simulink model "torqueBalancingJc"  (Simulink 8.6)
settings: Solver=FixedStepDiscrete  StartTime=0.0  StopTime=simulationTime  FixedStep=Ts  RelTol=1e-3
InitFcn:
  | initTorqueBalancingJc;
values from neighbouring files (symbols this model uses):
  LEFT_RIGHT_FOOT_IN_CONTACT = [1 1]    [initTorqueBalancingJc.m]
  localName = 'matlabTorqueBalancing'    [initTorqueBalancingJc.m]
  Ts = 0.01    [initTorqueBalancingJc.m]
undefined symbols (not defined in the file or in its folder): bVectorConstraints, ConstraintsMatrix, gain, impedencesSat, reg, ROBOT_DOF, ROBOT_DOF_FOR_SIMULINK, sat
undefined symbols (not defined in the file): robotName
libraries: WBCLibrary x63, simulink x2
settings Model: Creator=daniele  LastModifiedBy=DanielePucci
settings DataIOCC: SignalLoggingSaveFormat=Dataset
settings DebuggingCC: FcnCallInpInsideContextMsg=EnableAllAsWarning
settings SFSimCC: SimParseCustomCode=off
settings ConfigComp: CovSFcnEnable=off

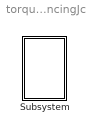
== system torqueBalancingJc ==
  Subsystem : Subsystem  mask{robotName=robotName, Ts=Ts, localName=localName}
      mask prompts: robotName "robot name"; localName "module name"

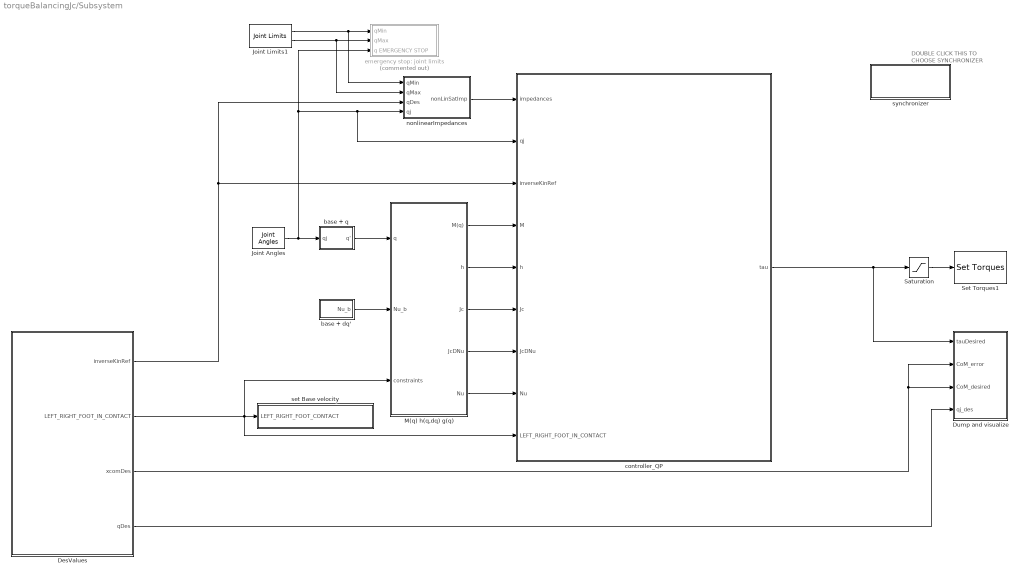
== system torqueBalancingJc/Subsystem ==
  note: DOUBLE CLICK THIS TO
      |  CHOOSE SYNCHRONIZER
  DesValues : Subsystem
  Dump and visualize : Subsystem
  Joint Angles : WBCLibrary/wholeBodyStates/Joint Angles  robotName=robotName  localName=localName
  Joint Limits1 : WBCLibrary/wholeBodyModel/Joint Limits  robotName=robotName  localName=localName
  M(q) h(q,dq) g(q) : Subsystem
  Saturation : Saturate  UpperLimit=sat.torque  LowerLimit=-sat.torque
  Set Torques1 : WBCLibrary/wholeBodyActuators/Set Torques  val=6  robotName=robotName  localName=localName
  base + dq' : Subsystem
  base + q : Subsystem
  controller_QP : Subsystem
  emergency stop: joint limits : Subsystem  Commented=on
  nonlinearImpedances : Subsystem
  set Base velocity : Subsystem  Description=Set base velocity
  synchronizer : Subsystem
  wires:
  base + q/1(q') -> M(q) h(q,dq) g(q)/1(q)
  base + dq'/1(Nu_b) -> M(q) h(q,dq) g(q)/2(Nu_b)
  M(q) h(q,dq) g(q)/1(M(q)) -> controller_QP/4(M)
  Joint Limits1/1 -> emergency stop: joint limits/1(qMin), nonlinearImpedances/1(qMin)
  Joint Limits1/2 -> emergency stop: joint limits/2(qMax), nonlinearImpedances/2(qMax)
  Joint Angles/1 -> emergency stop: joint limits/3(q EMERGENCY STOP), controller_QP/2(qj), nonlinearImpedances/4(qj), base + q/1(qj)
  M(q) h(q,dq) g(q)/2(h) -> controller_QP/5(h)
  controller_QP/1("tau ") -> Dump and visualize/1(tauDesired), Saturation/1
  Saturation/1 -> Set Torques1/1
  DesValues/2(LEFT_RIGHT_FOOT_IN_CONTACT) -> M(q) h(q,dq) g(q)/3(constraints), set Base velocity/1(LEFT_RIGHT_FOOT_CONTACT), controller_QP/9(LEFT_RIGHT_FOOT_IN_CONTACT)
  DesValues/3(xcomDes) -> Dump and visualize/2(CoM_error), Dump and visualize/3(CoM_desired)
  nonlinearImpedances/1(nonLinSatImp) -> controller_QP/1(impedances)
  M(q) h(q,dq) g(q)/5(Nu) -> controller_QP/8(Nu)
  M(q) h(q,dq) g(q)/3(Jc) -> controller_QP/6(Jc)
  M(q) h(q,dq) g(q)/4(JcDNu) -> controller_QP/7(JcDNu)
  DesValues/1(inverseKinRef) -> nonlinearImpedances/3(qDes), controller_QP/3(inverseKinRef)
  DesValues/4(qDes) -> Dump and visualize/4(qj_des)

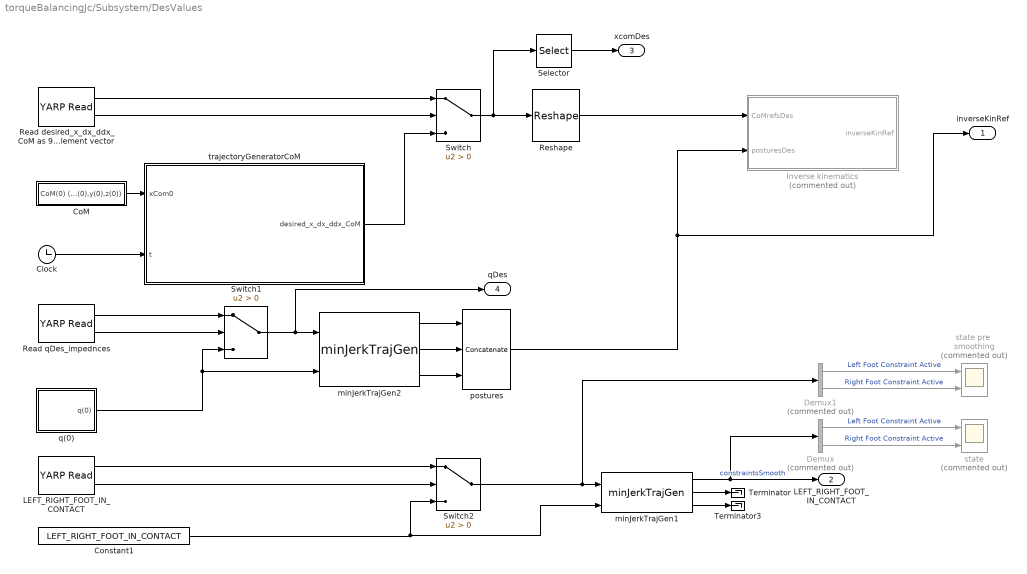
== system torqueBalancingJc/Subsystem/DesValues ==
  " LEFT_RIGHT_FOOT_IN_CONTACT" : WBCLibrary/Utilities/YARP Read  portName=['/' localName '/constraints:i']  signalSize=2  blocking=off  timestamp=off  autoconnect=off  errorOnConnection=on
  Clock : Clock
  "CoM " : Subsystem
  Constant1 : Constant  Value=LEFT_RIGHT_FOOT_IN_CONTACT
  Demux : Demux  Commented=on  Outputs=2
  Demux1 : Demux  Commented=on  Outputs=2
  Inverse kinematics : Subsystem  Commented=on
  "Read desired_x_dx_ddx_CoM as 9 element vector " : WBCLibrary/Utilities/YARP Read  portName=['/' localName '/comDes:i']  signalSize=9  blocking=off  timestamp=off  autoconnect=off  errorOnConnection=on
  Read qDes_impednces : WBCLibrary/Utilities/YARP Read  portName=['/' localName '/qDes:i']  signalSize=ROBOT_DOF  blocking=off  timestamp=off  autoconnect=off  errorOnConnection=on
  Reshape : Reshape  OutputDimensionality=Customize  OutputDimensions=[3,3]
  Selector : Selector  InputPortWidth=9  IndexOptions=Index vector (dialog)  Indices=[1:3]  OutputSizes=1
  Switch : Switch  Criteria=u2 > Threshold
  Switch1 : Switch  Criteria=u2 > Threshold
  Switch2 : Switch  Criteria=u2 > Threshold
  Terminator : Terminator
  Terminator3 : Terminator
  minJerkTrajGen1 : WBCLibrary/Utilities/minJerkTrajGen  dim=2  Ts=Ts  Tt=smoothingTimeJacobians
  minJerkTrajGen2 : WBCLibrary/Utilities/minJerkTrajGen  dim=ROBOT_DOF  Ts=Ts  Tt=smoothingTimePostures
  postures : Concatenate  NumInputs=3  Mode=Multidimensional array  ConcatenateDimension=2
  q(0) : Subsystem
  state : Scope  Commented=on  NumInputPorts=2
  state pre  smoothing : Scope  Commented=on  NumInputPorts=2
  trajectoryGeneratorCoM : MATLAB Function  TreatAsAtomicUnit=on
  inverseKinRef : Outport
  LEFT_RIGHT_FOOT_IN_CONTACT : Outport  Port=2
  xcomDes : Outport  Port=3
  qDes : Outport  Port=4
  wires:
  Constant1/1 -> minJerkTrajGen1/2, Switch2/3
  minJerkTrajGen1/1 -> Demux/1, LEFT_RIGHT_FOOT_IN_CONTACT/1  "constraintsSmooth"
  minJerkTrajGen1/2 -> Terminator/1
  minJerkTrajGen1/3 -> Terminator3/1
  "Read desired_x_dx_ddx_CoM as 9 element vector "/2 -> Switch/2
  "Read desired_x_dx_ddx_CoM as 9 element vector "/1 -> Switch/1
  Reshape/1 -> Inverse kinematics/1(CoMrefsDes)
  Switch/1 -> Selector/1, Reshape/1
  Read qDes_impednces/2 -> Switch1/2
  Read qDes_impednces/1 -> Switch1/1
  q(0)/1(q(0)) -> Switch1/3, minJerkTrajGen2/2
  Selector/1 -> xcomDes/1
  " LEFT_RIGHT_FOOT_IN_CONTACT"/2 -> Switch2/2
  " LEFT_RIGHT_FOOT_IN_CONTACT"/1 -> Switch2/1
  Switch2/1 -> Demux1/1, minJerkTrajGen1/1
  Demux/1 -> state/1  "Left Foot Constraint Active"
  Demux/2 -> state/2  "Right Foot Constraint Active"
  Demux1/1 -> state pre  smoothing/1  "Left Foot Constraint Active"
  Demux1/2 -> state pre  smoothing/2  "Right Foot Constraint Active"
  "CoM "/1(CoM(0) (x(0),y(0),z(0))) -> trajectoryGeneratorCoM/1(xCom0)
  Clock/1 -> trajectoryGeneratorCoM/2(t)
  trajectoryGeneratorCoM/1(desired_x_dx_ddx_CoM) -> Switch/3
  Switch1/1 -> qDes/1, minJerkTrajGen2/1
  minJerkTrajGen2/1 -> postures/1
  minJerkTrajGen2/2 -> postures/2
  minJerkTrajGen2/3 -> postures/3
  postures/1 -> inverseKinRef/1, Inverse kinematics/2(posturesDes)

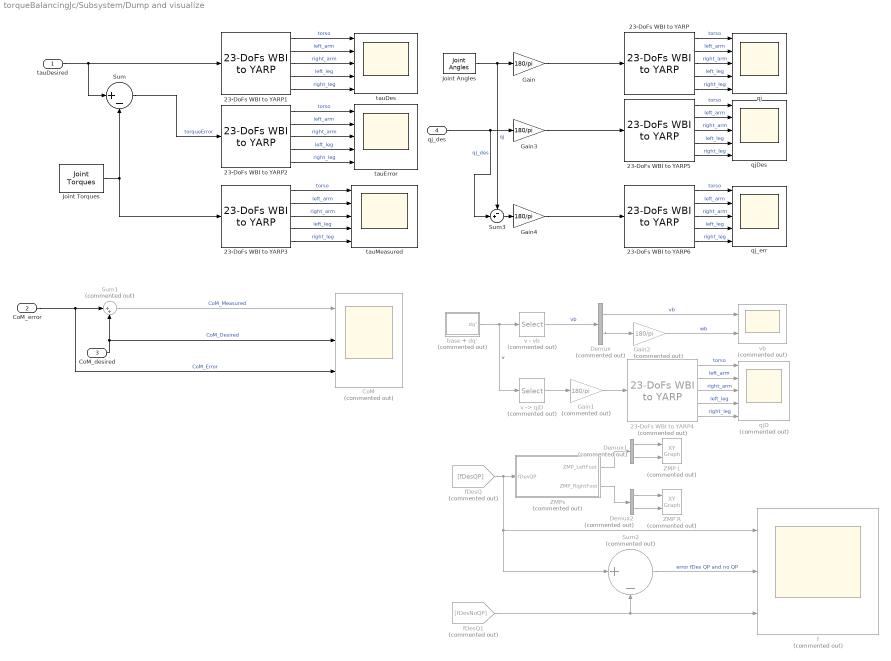
== system torqueBalancingJc/Subsystem/Dump and visualize ==
  tauDesired : Inport
  CoM_error : Inport  Port=2
  CoM_desired : Inport  Port=3
  qj_des : Inport  Port=4
  23-DoFs WBI to YARP{,1..3,5..6} (6 alike) : WBCLibrary/Utilities/23-DoFs WBI to YARP
  23-DoFs WBI to YARP4 : WBCLibrary/Utilities/23-DoFs WBI to YARP  Commented=on
  CoM : Scope  Commented=on  NumInputPorts=3
  Demux : Demux  Commented=on  Outputs=2
  Demux1 : Demux  Commented=on  Outputs=2
  Demux2 : Demux  Commented=on  Outputs=2
  Gain : Gain  Gain=180/pi
  Gain1 : Gain  Commented=on  Gain=180/pi
  Gain2 : Gain  Commented=on  Gain=180/pi
  Gain3 : Gain  Gain=180/pi
  Gain4 : Gain  Gain=180/pi
  Joint Angles : WBCLibrary/wholeBodyStates/Joint Angles  robotName=robotName  localName=localName
  Joint Torques : WBCLibrary/wholeBodyStates/Joint Torques  robotName=robotName  localName=localName
  Sum : Sum  Inputs=|+-
  Sum1 : Sum  Commented=on  Inputs=|++
  Sum2 : Sum  Commented=on  Inputs=|+-
  Sum3 : Sum  Inputs=-+|
  ZMP L : simulink/Sinks/XY Graph  Commented=on  xmin=gain.footSize(1,1)  xmax=gain.footSize(1,2)  ymin=gain.footSize(2,1)  ymax=gain.footSize(2,2)  st=-1
  ZMP R : simulink/Sinks/XY Graph  Commented=on  xmin=gain.footSize(1,1)  xmax=gain.footSize(1,2)  ymin=gain.footSize(2,1)  ymax=gain.footSize(2,2)  st=-1
  ZMPs : Subsystem  Commented=on
  base + dq' : Subsystem  Commented=on
  f : Scope  Commented=on  NumInputPorts=3
  fDesQ : From  Commented=on  GotoTag=fDesQP  TagVisibility=global
  fDesQ1 : From  Commented=on  GotoTag=fDesNoQP  TagVisibility=global
  qj : Scope  NumInputPorts=5
  qjD : Scope  Commented=on  NumInputPorts=5
  qjDes : Scope  NumInputPorts=5
  qj_err : Scope  NumInputPorts=5
  tauDes : Scope  NumInputPorts=5
  tauError : Scope  NumInputPorts=5
  tauMeasured : Scope  NumInputPorts=5
  v - vb : Selector  Commented=on  InputPortWidth=ROBOT_DOF+6  IndexOptions=Index vector (dialog)  Indices=[1:6]  OutputSizes=1
  "v -> qjD" : Selector  Commented=on  InputPortWidth=ROBOT_DOF+6  IndexOptions=Index vector (dialog)  Indices=[7:ROBOT_DOF+6]  OutputSizes=1
  vb : Scope  Commented=on  NumInputPorts=2
  wires:
  CoM_error/1 -> CoM/3, Sum1/1  "CoM_Error"
  CoM_desired/1 -> Sum1/2, CoM/2  "CoM_Desired"
  Sum1/1 -> CoM/1  "CoM_Measured"
  base + dq'/1(dq') -> "v -> qjD"/1, v - vb/1  "v"
  Joint Angles/1 -> Sum3/1, Gain/1  "qj"
  Gain/1 -> 23-DoFs WBI to YARP/1
  23-DoFs WBI to YARP/5 -> qj/5  "right_leg"
  23-DoFs WBI to YARP/1 -> qj/1  "torso"
  23-DoFs WBI to YARP/2 -> qj/2  "left_arm"
  23-DoFs WBI to YARP/4 -> qj/4  "left_leg"
  23-DoFs WBI to YARP/3 -> qj/3  "right_arm"
  23-DoFs WBI to YARP4/5 -> qjD/5  "right_leg"
  23-DoFs WBI to YARP4/1 -> qjD/1  "torso"
  23-DoFs WBI to YARP4/2 -> qjD/2  "left_arm"
  23-DoFs WBI to YARP4/4 -> qjD/4  "left_leg"
  23-DoFs WBI to YARP4/3 -> qjD/3  "right_arm"
  "v -> qjD"/1 -> Gain1/1
  v - vb/1 -> Demux/1  "vb"
  Demux/1 -> vb/1  "vb"
  Demux/2 -> Gain2/1
  Gain1/1 -> 23-DoFs WBI to YARP4/1
  Gain2/1 -> vb/2  "wb"
  fDesQ/1 -> Sum2/1, f/1, ZMPs/1(fDesQP)
  ZMPs/1(ZMP_LeftFoot) -> Demux1/1
  ZMPs/2(ZMP_RightFoot) -> Demux2/1
  Demux1/1 -> ZMP L/1
  Demux1/2 -> ZMP L/2
  Demux2/1 -> ZMP R/1
  Demux2/2 -> ZMP R/2
  Sum2/1 -> f/2  "error fDes QP and no QP"
  fDesQ1/1 -> Sum2/2, f/3
  tauDesired/1 -> Sum/1, 23-DoFs WBI to YARP1/1
  Joint Torques/1 -> 23-DoFs WBI to YARP3/1, Sum/2
  23-DoFs WBI to YARP1/5 -> tauDes/5  "right_leg"
  23-DoFs WBI to YARP1/1 -> tauDes/1  "torso"
  23-DoFs WBI to YARP1/2 -> tauDes/2  "left_arm"
  23-DoFs WBI to YARP1/4 -> tauDes/4  "left_leg"
  23-DoFs WBI to YARP1/3 -> tauDes/3  "right_arm"
  23-DoFs WBI to YARP2/5 -> tauError/5  "right_leg"
  23-DoFs WBI to YARP2/1 -> tauError/1  "torso"
  23-DoFs WBI to YARP2/2 -> tauError/2  "left_arm"
  23-DoFs WBI to YARP2/4 -> tauError/4  "left_leg"
  23-DoFs WBI to YARP2/3 -> tauError/3  "right_arm"
  Sum/1 -> 23-DoFs WBI to YARP2/1  "torqueError"
  23-DoFs WBI to YARP3/5 -> tauMeasured/5  "right_leg"
  23-DoFs WBI to YARP3/1 -> tauMeasured/1  "torso"
  23-DoFs WBI to YARP3/2 -> tauMeasured/2  "left_arm"
  23-DoFs WBI to YARP3/4 -> tauMeasured/4  "left_leg"
  23-DoFs WBI to YARP3/3 -> tauMeasured/3  "right_arm"
  Gain3/1 -> 23-DoFs WBI to YARP5/1
  23-DoFs WBI to YARP5/5 -> qjDes/5  "right_leg"
  23-DoFs WBI to YARP5/1 -> qjDes/1  "torso"
  23-DoFs WBI to YARP5/2 -> qjDes/2  "left_arm"
  23-DoFs WBI to YARP5/4 -> qjDes/4  "left_leg"
  23-DoFs WBI to YARP5/3 -> qjDes/3  "right_arm"
  Gain4/1 -> 23-DoFs WBI to YARP6/1
  23-DoFs WBI to YARP6/5 -> qj_err/5  "right_leg"
  23-DoFs WBI to YARP6/1 -> qj_err/1  "torso"
  23-DoFs WBI to YARP6/2 -> qj_err/2  "left_arm"
  23-DoFs WBI to YARP6/4 -> qj_err/4  "left_leg"
  23-DoFs WBI to YARP6/3 -> qj_err/3  "right_arm"
  Sum3/1 -> Gain4/1
  qj_des/1 -> Sum3/2, Gain3/1  "qj_des"

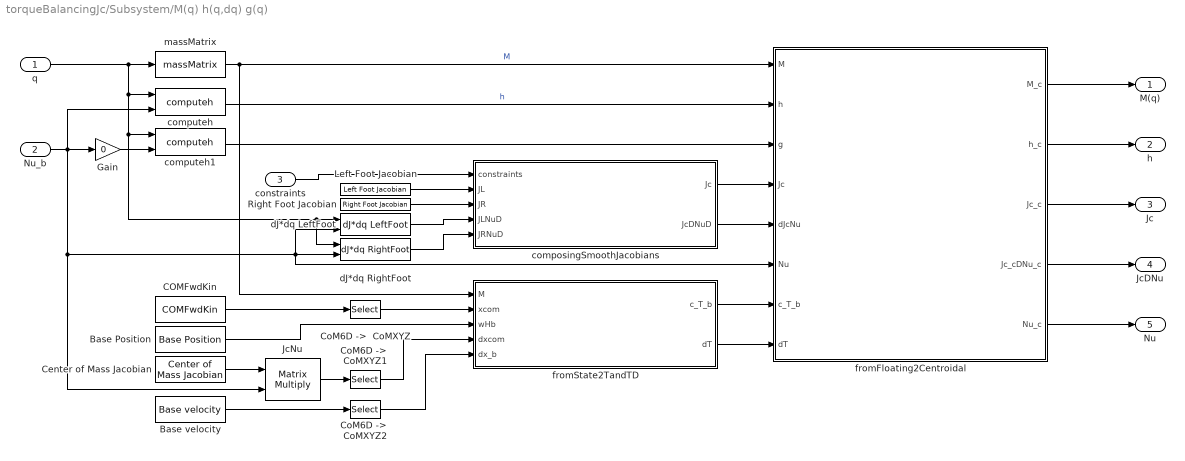
== system torqueBalancingJc/Subsystem/M(q) h(q,dq) g(q) ==
  q : Inport
  Nu_b : Inport  Port=2
  constraints : Inport  Port=3
  Base Position : WBCLibrary/wholeBodyStates/Base Position  robotName=robotName  localName=localName
  Base velocity : WBCLibrary/wholeBodyStates/Base velocity  robotName=robotName  localName=localName
  "COMFwdKin " : WBCLibrary/wholeBodyModel/Forward Kinematics/COMFwdKin   robotName=robotName  localName=localName
  Center of Mass Jacobian : WBCLibrary/wholeBodyModel/Jacobians/Center of Mass Jacobian  robotName=robotName  localName=localName
  "CoM6D ->  CoMXYZ" : Selector  InputPortWidth=7  IndexOptions=Index vector (dialog)  Indices=[1 2 3]  OutputSizes=1
  "CoM6D ->  CoMXYZ1" : Selector  InputPortWidth=6  IndexOptions=Index vector (dialog)  Indices=[1 2 3]  OutputSizes=1
  "CoM6D ->  CoMXYZ2" : Selector  InputPortWidth=6  IndexOptions=Index vector (dialog)  Indices=[1 2 3]  OutputSizes=1
  Gain : Gain  Gain=0
  JcNu : Product  Multiplication=Matrix(*)
  Left Foot Jacobian : WBCLibrary/wholeBodyModel/Jacobians/Left Foot Jacobian  robotName=robotName  localName=localName
  Right Foot Jacobian : WBCLibrary/wholeBodyModel/Jacobians/Right Foot Jacobian  robotName=robotName  localName=localName
  composingSmoothJacobians : MATLAB Function  TreatAsAtomicUnit=on
  computeh : WBCLibrary/wholeBodyModel/Dynamics/computeh  val=7  robotname=robotName  localname=localName
  computeh1 : WBCLibrary/wholeBodyModel/Dynamics/computeh  val=7  robotname=robotName  localname=localName
  dJ*dq LeftFoot : WBCLibrary/wholeBodyModel/Dynamics/dJ*dq LeftFoot  val=9  robotName=robotName  localName=localName
  dJ*dq RightFoot : WBCLibrary/wholeBodyModel/Dynamics/dJ*dq RightFoot  val=9  robotName=robotName  localName=localName
  fromFloating2Centroidal : MATLAB Function  TreatAsAtomicUnit=on
  fromState2TandTD : MATLAB Function  TreatAsAtomicUnit=on
  massMatrix : WBCLibrary/wholeBodyModel/Dynamics/massMatrix  val=8  robotname=robotName  localname=localName
  M(q) : Outport
  h : Outport  Port=2
  Jc : Outport  Port=3
  JcDNu : Outport  Port=4
  Nu : Outport  Port=5
  wires:
  q/1 -> computeh1/1, dJ*dq RightFoot/1, dJ*dq LeftFoot/1, computeh/1, massMatrix/1
  Nu_b/1 -> Gain/1, computeh/2, fromFloating2Centroidal/6(Nu), dJ*dq LeftFoot/2, dJ*dq RightFoot/2, JcNu/2
  Gain/1 -> computeh1/2
  massMatrix/1 -> fromFloating2Centroidal/1(M), fromState2TandTD/1(M)  "M"
  fromState2TandTD/1(c_T_b) -> fromFloating2Centroidal/7(c_T_b)
  fromState2TandTD/2(dT) -> fromFloating2Centroidal/8(dT)
  computeh/1 -> fromFloating2Centroidal/2(h)  "h"
  computeh1/1 -> fromFloating2Centroidal/3(g)
  "COMFwdKin "/1 -> "CoM6D ->  CoMXYZ"/1
  "CoM6D ->  CoMXYZ"/1 -> fromState2TandTD/2(xcom)
  Base velocity/1 -> "CoM6D ->  CoMXYZ2"/1
  "CoM6D ->  CoMXYZ2"/1 -> fromState2TandTD/5(dx_b)
  Base Position/1 -> fromState2TandTD/3(wHb)
  Center of Mass Jacobian/1 -> JcNu/1
  JcNu/1 -> "CoM6D ->  CoMXYZ1"/1
  "CoM6D ->  CoMXYZ1"/1 -> fromState2TandTD/4(dxcom)
  composingSmoothJacobians/1(Jc) -> fromFloating2Centroidal/4(Jc)
  composingSmoothJacobians/2(JcDNuD) -> fromFloating2Centroidal/5(dJcNu)
  constraints/1 -> composingSmoothJacobians/1(constraints)
  Left Foot Jacobian/1 -> composingSmoothJacobians/2(JL)
  Right Foot Jacobian/1 -> composingSmoothJacobians/3(JR)
  dJ*dq LeftFoot/1 -> composingSmoothJacobians/4(JLNuD)
  dJ*dq RightFoot/1 -> composingSmoothJacobians/5(JRNuD)
  fromFloating2Centroidal/1(M_c) -> M(q)/1
  fromFloating2Centroidal/2(h_c) -> h/1
  fromFloating2Centroidal/3(Jc_c) -> Jc/1
  fromFloating2Centroidal/4(Jc_cDNu_c) -> JcDNu/1
  fromFloating2Centroidal/5(Nu_c) -> Nu/1

== system torqueBalancingJc/Subsystem/base + dq' ==
  Base velocity : WBCLibrary/wholeBodyStates/Base velocity  robotName=robotName  localName=localName
  Joint Velocities : WBCLibrary/wholeBodyStates/Joint Velocities  robotName=robotName  localName=localName
  Mux : Mux  Inputs=2
  Nu_b : Outport
  wires:
  Base velocity/1 -> Mux/1
  Joint Velocities/1 -> Mux/2
  Mux/1 -> Nu_b/1

== system torqueBalancingJc/Subsystem/base + q ==
  qj : Inport
  Constant1 : Constant  Value=zeros(16,1)
  Mux : Mux  Inputs=2
  q' : Outport
  wires:
  Mux/1 -> q'/1
  qj/1 -> Mux/2
  Constant1/1 -> Mux/1

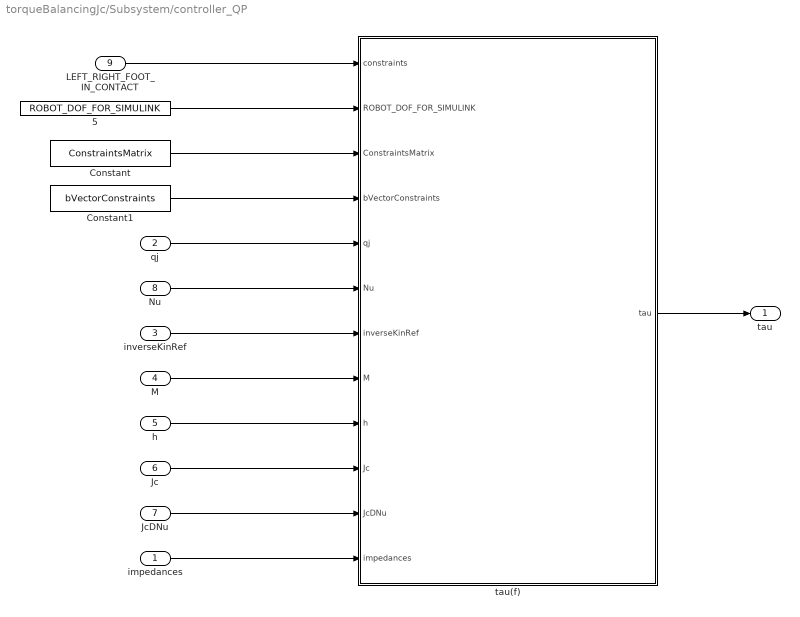
== system torqueBalancingJc/Subsystem/controller_QP ==
  impedances : Inport
  qj : Inport  Port=2
  inverseKinRef : Inport  Port=3
  M : Inport  Port=4
  h : Inport  Port=5
  Jc : Inport  Port=6
  JcDNu : Inport  Port=7
  Nu : Inport  Port=8
  LEFT_RIGHT_FOOT_IN_CONTACT : Inport  Port=9
  "    5" : Constant  Value=ROBOT_DOF_FOR_SIMULINK
  Constant : Constant  Value=ConstraintsMatrix
  Constant1 : Constant  Value=bVectorConstraints
  "tau(f) " : MATLAB Function  TreatAsAtomicUnit=on
  "tau " : Outport
  wires:
  LEFT_RIGHT_FOOT_IN_CONTACT/1 -> "tau(f) "/1(constraints)
  M/1 -> "tau(f) "/8(M)
  h/1 -> "tau(f) "/9(h)
  "    5"/1 -> "tau(f) "/2(ROBOT_DOF_FOR_SIMULINK)
  Constant/1 -> "tau(f) "/3(ConstraintsMatrix)
  Constant1/1 -> "tau(f) "/4(bVectorConstraints)
  Jc/1 -> "tau(f) "/10(Jc)
  JcDNu/1 -> "tau(f) "/11(JcDNu)
  Nu/1 -> "tau(f) "/6(Nu)
  impedances/1 -> "tau(f) "/12(impedances)
  "tau(f) "/1(tau) -> "tau "/1
  qj/1 -> "tau(f) "/5(qj)
  inverseKinRef/1 -> "tau(f) "/7(inverseKinRef)

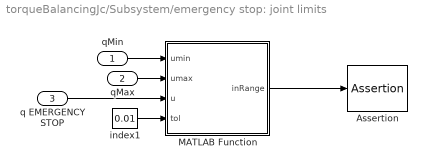
== system torqueBalancingJc/Subsystem/emergency stop: joint limits ==
  qMin : Inport
  qMax : Inport  Port=2
  q EMERGENCY STOP : Inport  Port=3
  Assertion : Assertion
  MATLAB Function : MATLAB Function  TreatAsAtomicUnit=on
  index1 : Constant  Value=0.01  VectorParams1D=off
  wires:
  qMin/1 -> MATLAB Function/1(umin)
  qMax/1 -> MATLAB Function/2(umax)
  index1/1 -> MATLAB Function/4(tol)
  q EMERGENCY STOP/1 -> MATLAB Function/3(u)
  MATLAB Function/1(inRange) -> Assertion/1

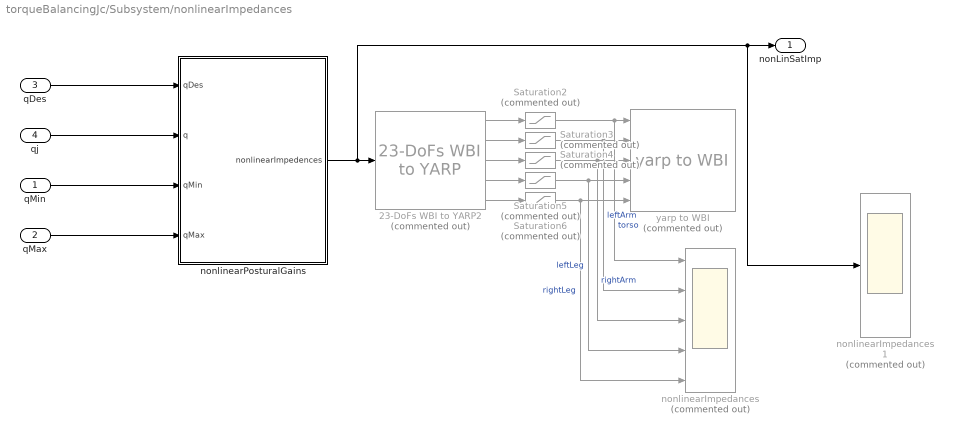
== system torqueBalancingJc/Subsystem/nonlinearImpedances ==
  qMin : Inport
  qMax : Inport  Port=2
  qDes : Inport  Port=3
  qj : Inport  Port=4
  23-DoFs WBI to YARP2 : WBCLibrary/Utilities/23-DoFs WBI to YARP  Commented=on
  Saturation2 : Saturate  Commented=on  UpperLimit=impedencesSat(1)  LowerLimit=0  SampleTime=Ts
  Saturation3 : Saturate  Commented=on  UpperLimit=impedencesSat(2)  LowerLimit=0  SampleTime=Ts
  Saturation4 : Saturate  Commented=on  UpperLimit=impedencesSat(2)  LowerLimit=0  SampleTime=Ts
  Saturation5 : Saturate  Commented=on  UpperLimit=impedencesSat(3)  LowerLimit=0  SampleTime=Ts
  Saturation6 : Saturate  Commented=on  UpperLimit=impedencesSat(3)  LowerLimit=0  SampleTime=Ts
  nonlinearImpedances : Scope  Commented=on  NumInputPorts=5
  nonlinearImpedances1 : Scope  Commented=on
  "nonlinearPosturalGains " : MATLAB Function  TreatAsAtomicUnit=on
  yarp to WBI : WBCLibrary/Utilities/yarp to WBI  Commented=on
  nonLinSatImp : Outport
  wires:
  23-DoFs WBI to YARP2/1 -> Saturation2/1
  23-DoFs WBI to YARP2/2 -> Saturation3/1
  23-DoFs WBI to YARP2/3 -> Saturation4/1
  23-DoFs WBI to YARP2/5 -> Saturation6/1
  "nonlinearPosturalGains "/1(nonlinearImpedences) -> nonlinearImpedances1/1, nonLinSatImp/1, 23-DoFs WBI to YARP2/1
  qMin/1 -> "nonlinearPosturalGains "/3(qMin)
  qMax/1 -> "nonlinearPosturalGains "/4(qMax)
  qj/1 -> "nonlinearPosturalGains "/2(q)
  Saturation6/1 -> nonlinearImpedances/5, yarp to WBI/5  "rightLeg"
  Saturation4/1 -> nonlinearImpedances/3, yarp to WBI/3  "rightArm"
  Saturation5/1 -> nonlinearImpedances/4, yarp to WBI/4  "leftLeg"
  Saturation3/1 -> nonlinearImpedances/2, yarp to WBI/2  "leftArm"
  Saturation2/1 -> nonlinearImpedances/1, yarp to WBI/1  "torso"
  23-DoFs WBI to YARP2/4 -> Saturation5/1
  qDes/1 -> "nonlinearPosturalGains "/1(qDes)

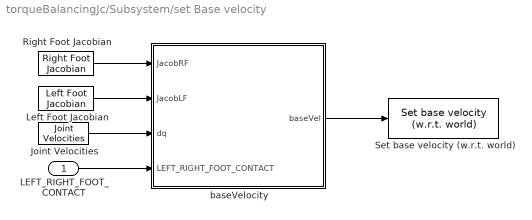
== system torqueBalancingJc/Subsystem/set Base velocity ==
  LEFT_RIGHT_FOOT_CONTACT : Inport
  Joint Velocities : WBCLibrary/wholeBodyStates/Joint Velocities  robotName=robotName  localName=localName
  Left Foot Jacobian : WBCLibrary/wholeBodyModel/Jacobians/Left Foot Jacobian  robotName=robotName  localName=localName
  Right Foot Jacobian : WBCLibrary/wholeBodyModel/Jacobians/Right Foot Jacobian  robotName=robotName  localName=localName
  Set base velocity (w.r.t. world) : WBCLibrary/wholeBodyStates/Set base velocity (w.r.t. world)  Priority=-1  robotName=robotName  localName=localName
  baseVelocity : Subsystem  AncestorBlock=WBCLibrary/Utilities/baseVelocity  mask(baseVelocity){}
      mask help: This block computes the velocity of the floating base of a bipedal robot
  wires:
  Left Foot Jacobian/1 -> baseVelocity/2(JacobLF)
  Right Foot Jacobian/1 -> baseVelocity/1(JacobRF)
  baseVelocity/1(baseVel) -> Set base velocity (w.r.t. world)/1
  Joint Velocities/1 -> baseVelocity/3(dq)
  LEFT_RIGHT_FOOT_CONTACT/1 -> baseVelocity/4(LEFT_RIGHT_FOOT_CONTACT)

== system torqueBalancingJc/Subsystem/synchronizer ==
  Real Time Synchronizer : WBCLibrary/Utilities/Real Time Synchronizer  threadPeriod=Ts
  synchronize : WBCLibrary/Utilities/synchronize  Commented=on  rate=0.010  scaleFactor=1

== system torqueBalancingJc/Subsystem/DesValues/CoM  ==
  "COMFwdKin " : WBCLibrary/wholeBodyModel/Forward Kinematics/COMFwdKin   robotName=robotName  localName=localName
  "CoM6D ->  CoMXYZ" : Selector  InputPortWidth=7  IndexOptions=Index vector (dialog)  Indices=[1 2 3]  OutputSizes=1
  "holder " : WBCLibrary/Utilities/holder 
  CoM(0) (x(0),y(0),z(0)) : Outport
  wires:
  "COMFwdKin "/1 -> "CoM6D ->  CoMXYZ"/1
  "CoM6D ->  CoMXYZ"/1 -> "holder "/1
  "holder "/1 -> CoM(0) (x(0),y(0),z(0))/1

== system torqueBalancingJc/Subsystem/DesValues/Inverse kinematics ==
  CoMrefsDes : Inport
  posturesDes : Inport  Port=2
  base + dq' : Subsystem
  iKin Stack of Tasks : Subsystem
  iKin correction terms : Subsystem
  inverseKinRef : Outport
  wires:
  CoMrefsDes/1 -> iKin correction terms/1(CoMrefsDes)
  posturesDes/1 -> iKin correction terms/2(posturesDes)
  base + dq'/1(Nu_b) -> iKin correction terms/4(Nu_iKin)

== system torqueBalancingJc/Subsystem/DesValues/q(0) ==
  Joint Angles : WBCLibrary/wholeBodyStates/Joint Angles  robotName=robotName  localName=localName
  holder 1 : WBCLibrary/Utilities/holder 
  q(0) : Outport
  wires:
  Joint Angles/1 -> holder 1/1
  holder 1/1 -> q(0)/1

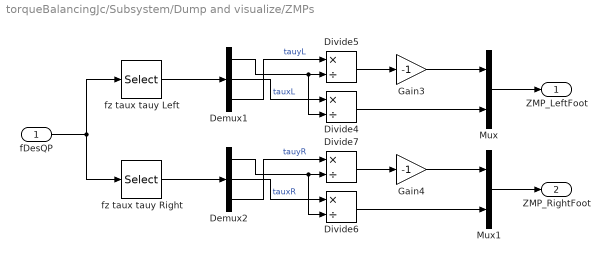
== system torqueBalancingJc/Subsystem/Dump and visualize/ZMPs ==
  fDesQP : Inport
  Demux1 : Demux  Outputs=3
  Demux2 : Demux  Outputs=3
  Divide{4..7} (4 alike) : Product  Inputs=*/
  Gain3 : Gain  Gain=-1
  Gain4 : Gain  Gain=-1
  Mux : Mux  Inputs=2
  Mux1 : Mux  Inputs=2
  fz taux tauy Left : Selector  InputPortWidth=12  IndexOptions=Index vector (dialog)  Indices=[3 4 5]  OutputSizes=1
  fz taux tauy Right : Selector  InputPortWidth=12  IndexOptions=Index vector (dialog)  Indices=[9 10 11]  OutputSizes=1
  ZMP_LeftFoot : Outport
  ZMP_RightFoot : Outport  Port=2
  wires:
  fz taux tauy Left/1 -> Demux1/1
  Demux1/1 -> Divide4/2, Divide5/2
  Divide7/1 -> Gain4/1
  Divide4/1 -> Mux/2
  Divide5/1 -> Gain3/1
  fz taux tauy Right/1 -> Demux2/1
  Demux2/1 -> Divide6/2, Divide7/2
  fDesQP/1 -> fz taux tauy Left/1, fz taux tauy Right/1
  Gain3/1 -> Mux/1
  Mux/1 -> ZMP_LeftFoot/1
  Divide6/1 -> Mux1/2
  Gain4/1 -> Mux1/1
  Mux1/1 -> ZMP_RightFoot/1
  Demux1/2 -> Divide4/1  "tauxL"
  Demux1/3 -> Divide5/1  "tauyL"
  Demux2/2 -> Divide6/1  "tauxR"
  Demux2/3 -> Divide7/1  "tauyR"

== system torqueBalancingJc/Subsystem/Dump and visualize/base + dq' ==
  Joint Velocities : WBCLibrary/wholeBodyStates/Joint Velocities  robotName=robotName  localName=localName
  Left Foot Jacobian : WBCLibrary/wholeBodyModel/Jacobians/Left Foot Jacobian  robotName=robotName  localName=localName
  Mux : Mux  Inputs=2
  Right Foot Jacobian : WBCLibrary/wholeBodyModel/Jacobians/Right Foot Jacobian  robotName=robotName  localName=localName
  baseVelocity : Subsystem  AncestorBlock=WBCLibrary/Utilities/baseVelocity  mask(baseVelocity){}
      mask help: This block computes the velocity of the floating base of a bipedal robot
  dq' : Outport
  wires:
  Left Foot Jacobian/1 -> baseVelocity/2(JacobLF)
  Right Foot Jacobian/1 -> baseVelocity/1(JacobRF)
  baseVelocity/1(baseVel) -> Mux/1
  Joint Velocities/1 -> baseVelocity/3(dq), Mux/2
  Mux/1 -> dq'/1

== system torqueBalancingJc/Subsystem/set Base velocity/baseVelocity ==
  JacobRF : Inport
  JacobLF : Inport  Port=2
  dq : Inport  Port=3
  LEFT_RIGHT_FOOT_CONTACT : Inport  Port=4
  MATLAB Function : MATLAB Function  TreatAsAtomicUnit=on
  baseVel : Outport
  wires:
  JacobLF/1 -> MATLAB Function/1(JcLeftFoot)
  JacobRF/1 -> MATLAB Function/2(JcRightFoot)
  MATLAB Function/1(y) -> baseVel/1
  dq/1 -> MATLAB Function/4(qD)
  LEFT_RIGHT_FOOT_CONTACT/1 -> MATLAB Function/3(activeFeetConstraints)

== system torqueBalancingJc/Subsystem/DesValues/Inverse kinematics/base + dq' ==
  Base velocity : WBCLibrary/wholeBodyStates/Base velocity  robotName=robotName  localName=localName
  Joint Velocities : WBCLibrary/wholeBodyStates/Joint Velocities  robotName=robotName  localName=localName
  Mux : Mux  Inputs=2
  Nu_b : Outport
  wires:
  Base velocity/1 -> Mux/1
  Joint Velocities/1 -> Mux/2
  Mux/1 -> Nu_b/1

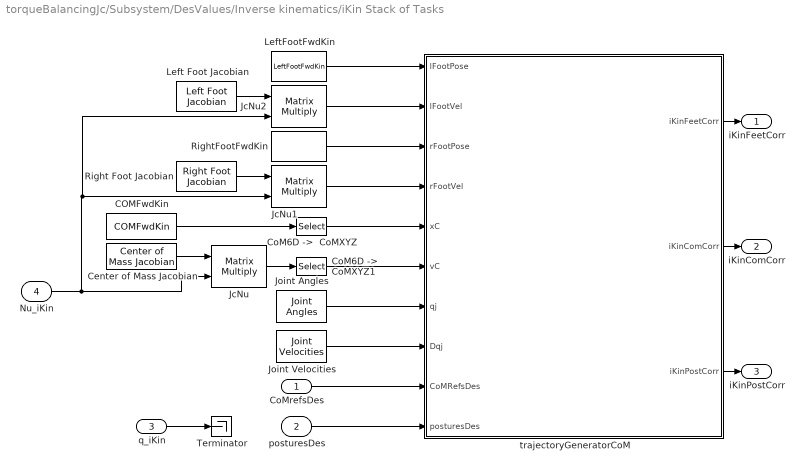
== system torqueBalancingJc/Subsystem/DesValues/Inverse kinematics/iKin Stack of Tasks ==
  CoMrefsDes : Inport
  posturesDes : Inport  Port=2
  q_iKin : Inport  Port=3
  Nu_iKin : Inport  Port=4
  "COMFwdKin " : WBCLibrary/wholeBodyModel/Forward Kinematics/COMFwdKin   robotName=robotName  localName=localName
  Center of Mass Jacobian : WBCLibrary/wholeBodyModel/Jacobians/Center of Mass Jacobian  robotName=robotName  localName=localName
  "CoM6D ->  CoMXYZ" : Selector  InputPortWidth=7  IndexOptions=Index vector (dialog)  Indices=[1 2 3]  OutputSizes=1
  "CoM6D ->  CoMXYZ1" : Selector  InputPortWidth=6  IndexOptions=Index vector (dialog)  Indices=[1 2 3]  OutputSizes=1
  JcNu : Product  Multiplication=Matrix(*)
  JcNu1 : Product  Multiplication=Matrix(*)
  JcNu2 : Product  Multiplication=Matrix(*)
  Joint Angles : WBCLibrary/wholeBodyStates/Joint Angles  robotName=robotName  localName=localName
  Joint Velocities : WBCLibrary/wholeBodyStates/Joint Velocities  robotName=robotName  localName=localName
  Left Foot Jacobian : WBCLibrary/wholeBodyModel/Jacobians/Left Foot Jacobian  robotName=robotName  localName=localName
  LeftFootFwdKin : WBCLibrary/wholeBodyModel/Forward Kinematics/LeftFootFwdKin  robotName=robotName  localName=localName
  Right Foot Jacobian : WBCLibrary/wholeBodyModel/Jacobians/Right Foot Jacobian  robotName=robotName  localName=localName
  RightFootFwdKin : WBCLibrary/wholeBodyModel/Forward Kinematics/RightFootFwdKin  robotName=robotName  localName=localName
  Terminator : Terminator
  trajectoryGeneratorCoM : MATLAB Function  TreatAsAtomicUnit=on
  iKinFeetCorr : Outport
  iKinComCorr : Outport  Port=2
  iKinPostCorr : Outport  Port=3
  wires:
  trajectoryGeneratorCoM/1(iKinFeetCorr) -> iKinFeetCorr/1
  trajectoryGeneratorCoM/3(iKinPostCorr) -> iKinPostCorr/1
  trajectoryGeneratorCoM/2(iKinComCorr) -> iKinComCorr/1
  CoMrefsDes/1 -> trajectoryGeneratorCoM/9(CoMRefsDes)
  "COMFwdKin "/1 -> "CoM6D ->  CoMXYZ"/1
  "CoM6D ->  CoMXYZ"/1 -> trajectoryGeneratorCoM/5(xC)
  Center of Mass Jacobian/1 -> JcNu/1
  JcNu/1 -> "CoM6D ->  CoMXYZ1"/1
  posturesDes/1 -> trajectoryGeneratorCoM/10(posturesDes)
  Joint Angles/1 -> trajectoryGeneratorCoM/7(qj)
  "CoM6D ->  CoMXYZ1"/1 -> trajectoryGeneratorCoM/6(vC)
  Joint Velocities/1 -> trajectoryGeneratorCoM/8(Dqj)
  q_iKin/1 -> Terminator/1
  LeftFootFwdKin/1 -> trajectoryGeneratorCoM/1(lFootPose)
  Nu_iKin/1 -> JcNu2/2, JcNu1/2, JcNu/2
  Right Foot Jacobian/1 -> JcNu1/1
  JcNu1/1 -> trajectoryGeneratorCoM/4(rFootVel)
  RightFootFwdKin/1 -> trajectoryGeneratorCoM/3(rFootPose)
  JcNu2/1 -> trajectoryGeneratorCoM/2(lFootVel)
  Left Foot Jacobian/1 -> JcNu2/1

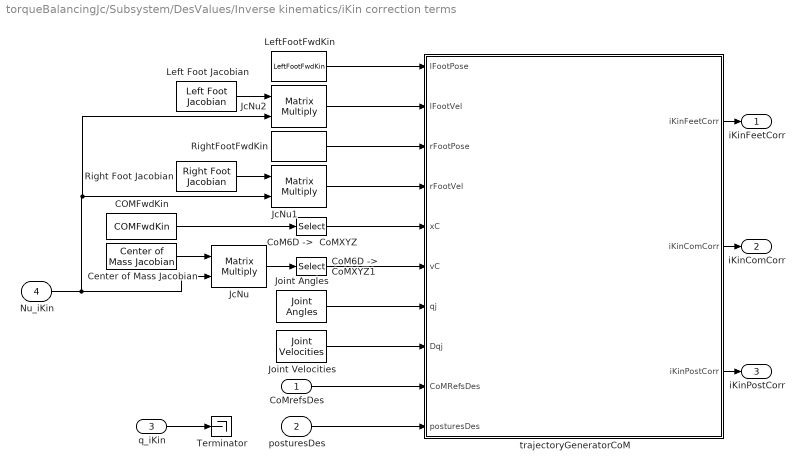
== system torqueBalancingJc/Subsystem/DesValues/Inverse kinematics/iKin correction terms ==
  CoMrefsDes : Inport
  posturesDes : Inport  Port=2
  q_iKin : Inport  Port=3
  Nu_iKin : Inport  Port=4
  "COMFwdKin " : WBCLibrary/wholeBodyModel/Forward Kinematics/COMFwdKin   robotName=robotName  localName=localName
  Center of Mass Jacobian : WBCLibrary/wholeBodyModel/Jacobians/Center of Mass Jacobian  robotName=robotName  localName=localName
  "CoM6D ->  CoMXYZ" : Selector  InputPortWidth=7  IndexOptions=Index vector (dialog)  Indices=[1 2 3]  OutputSizes=1
  "CoM6D ->  CoMXYZ1" : Selector  InputPortWidth=6  IndexOptions=Index vector (dialog)  Indices=[1 2 3]  OutputSizes=1
  JcNu : Product  Multiplication=Matrix(*)
  JcNu1 : Product  Multiplication=Matrix(*)
  JcNu2 : Product  Multiplication=Matrix(*)
  Joint Angles : WBCLibrary/wholeBodyStates/Joint Angles  robotName=robotName  localName=localName
  Joint Velocities : WBCLibrary/wholeBodyStates/Joint Velocities  robotName=robotName  localName=localName
  Left Foot Jacobian : WBCLibrary/wholeBodyModel/Jacobians/Left Foot Jacobian  robotName=robotName  localName=localName
  LeftFootFwdKin : WBCLibrary/wholeBodyModel/Forward Kinematics/LeftFootFwdKin  robotName=robotName  localName=localName
  Right Foot Jacobian : WBCLibrary/wholeBodyModel/Jacobians/Right Foot Jacobian  robotName=robotName  localName=localName
  RightFootFwdKin : WBCLibrary/wholeBodyModel/Forward Kinematics/RightFootFwdKin  robotName=robotName  localName=localName
  Terminator : Terminator
  trajectoryGeneratorCoM : MATLAB Function  TreatAsAtomicUnit=on
  iKinFeetCorr : Outport
  iKinComCorr : Outport  Port=2
  iKinPostCorr : Outport  Port=3
  wires:
  trajectoryGeneratorCoM/1(iKinFeetCorr) -> iKinFeetCorr/1
  trajectoryGeneratorCoM/3(iKinPostCorr) -> iKinPostCorr/1
  trajectoryGeneratorCoM/2(iKinComCorr) -> iKinComCorr/1
  CoMrefsDes/1 -> trajectoryGeneratorCoM/9(CoMRefsDes)
  "COMFwdKin "/1 -> "CoM6D ->  CoMXYZ"/1
  "CoM6D ->  CoMXYZ"/1 -> trajectoryGeneratorCoM/5(xC)
  Center of Mass Jacobian/1 -> JcNu/1
  JcNu/1 -> "CoM6D ->  CoMXYZ1"/1
  posturesDes/1 -> trajectoryGeneratorCoM/10(posturesDes)
  Joint Angles/1 -> trajectoryGeneratorCoM/7(qj)
  "CoM6D ->  CoMXYZ1"/1 -> trajectoryGeneratorCoM/6(vC)
  Joint Velocities/1 -> trajectoryGeneratorCoM/8(Dqj)
  LeftFootFwdKin/1 -> trajectoryGeneratorCoM/1(lFootPose)
  JcNu1/1 -> trajectoryGeneratorCoM/4(rFootVel)
  RightFootFwdKin/1 -> trajectoryGeneratorCoM/3(rFootPose)
  JcNu2/1 -> trajectoryGeneratorCoM/2(lFootVel)
  q_iKin/1 -> Terminator/1
  Nu_iKin/1 -> JcNu2/2, JcNu1/2, JcNu/2
  Left Foot Jacobian/1 -> JcNu2/1
  Right Foot Jacobian/1 -> JcNu1/1

== system torqueBalancingJc/Subsystem/Dump and visualize/base + dq'/baseVelocity ==
  JacobRF : Inport
  JacobLF : Inport  Port=2
  dq : Inport  Port=3
  Constant : Constant  Value=LEFT_RIGHT_FOOT_IN_CONTACT
  MATLAB Function : MATLAB Function  TreatAsAtomicUnit=on
  baseVel : Outport
  wires:
  JacobLF/1 -> MATLAB Function/1(JcLeftFoot)
  JacobRF/1 -> MATLAB Function/2(JcRightFoot)
  MATLAB Function/1(y) -> baseVel/1
  dq/1 -> MATLAB Function/4(qD)
  Constant/1 -> MATLAB Function/3(activeFeetConstraints)

== matlab function Subsystem/M(q) h(q,dq) g(q)/fromFloating2Centroidal ==
  data: M input double; M_c output double; h input double; g input double; Jc input double; dJcNu input double; Nu input double; c_T_b input double; dT input double; h_c output double; Jc_c output double; Jc_cDNu_c output double; Nu_c output double
function [M_c,h_c, Jc_c, Jc_cDNu_c, Nu_c] = fromFloating2Centroidal(M, h, g, Jc, dJcNu, Nu, c_T_b, dT)
%#codegen
[M_c,C_cNu_c, g_c, Jc_c, Jc_cDNu_c, Nu_c] = fromFloatingToCentroidalDynamics(M, h, g, Jc, dJcNu, Nu, c_T_b, dT);
h_c = C_cNu_c + g_c;

== matlab function Subsystem/DesValues/Inverse kinematics/iKin Stack of Tasks/trajectoryGeneratorCoM ==
  data: lFootPose input double; lFootVel input double; rFootPose input double; rFootVel input double; xC input double; vC input double; qj input double; Dqj input double; iKinFeetCorr output double; CoMRefsDes input double; iKinComCorr output double; iKinPostCorr output double; posturesDes input double; gain parameter double
function [iKinFeetCorr,iKinComCorr,iKinPostCorr]  = fcn(lFootPose,lFootVel,rFootPose,rFootVel,xC,vC,qj,Dqj,CoMRefsDes,posturesDes,gain)
%#codegen

iKinFeetCorr = [-gain.ikin.kp*lFootPose(1:3)-gain.ikin.kd*lFootVel(1:3);
                                            -gain.ikin.kd*lFootVel(4:6);
                -gain.ikin.kp*rFootPose(1:3)-gain.ikin.kd*rFootVel(1:3);
                                            -gain.ikin.kd*rFootVel(4:6)];
                                        
iKinComCorr  = CoMRefsDes(:,3)-gain.ikin.kp*(xC-CoMRefsDes(:,1))-gain.ikin.kd*(vC-CoMRefsDes(:,2));

iKinPostCorr = posturesDes(:,3)-gain.ikin.kp*(qj-posturesDes(:,1))-gain.ikin.kd*(Dqj-posturesDes(:,2));

== matlab function Subsystem/DesValues/trajectoryGeneratorCoM ==
  data: desired_x_dx_ddx_CoM output double; xCom0 input double; t input double; references parameter double
function desired_x_dx_ddx_CoM   = fcn(xCom0,t,references)
%#codegen
        
if t > references.noOscillationTime
    A = references.amplitudeOfOscillation;
else
    A = 0;
end
f = references.frequencyOfOscillation;

xcomDes    = xCom0 + A*sin(2*pi*f*t)*references.directionOfOscillation;
% xcomDes(1) =  xcomDes(1) + 0.01;
xDcomDes   =         A*2*pi*f*cos(2*pi*f*t)*references.directionOfOscillation;
xDDcomDes  =        -A*(2*pi*f)^2*sin(2*pi*f*t)*references.directionOfOscillation;

desired_x_dx_ddx_CoM = [xcomDes;xDcomDes;xDDcomDes];

== matlab function Subsystem/emergency stop: joint limits/MATLAB Function ==
  data: umin input double; umax input double; u input double; inRange output double; tol input double
function inRange = checkRange(umin, umax, u, tol)
%#codegen

res = u < umin + tol | u > umax - tol;
res = sum(res);
if res==0
    inRange = 1;
else
    inRange = 0;
    u < umin + tol | u > umax - tol
end

== matlab function Subsystem/controller_QP/tau(f)  ==
  data: tau output double; constraints input double; ROBOT_DOF_FOR_SIMULINK input double; ConstraintsMatrix input double; bVectorConstraints input double; qj input double; Nu input double; inverseKinRef input double; M input double; h input double; Jc input double; JcDNu input double; impedances input double; reg parameter double; gain parameter double
function tau    =  controller(constraints,ROBOT_DOF_FOR_SIMULINK,ConstraintsMatrix,bVectorConstraints,qj,Nu,inverseKinRef, M,h , Jc, JcDNu, impedances,reg,gain)
%#codegen

ROBOT_DOF = size(ROBOT_DOF_FOR_SIMULINK,1);

qTilde    = qj - inverseKinRef(:,1);
qTildeD   = Nu(7:end) - inverseKinRef(:,2);
qDesDD    = inverseKinRef(:,3);
tau       = controllerFCN(constraints, ROBOT_DOF, M, h, Jc, JcDNu,impedances, gain.dampings, qTilde,qTildeD, qDesDD,reg);

== matlab function Subsystem/M(q) h(q,dq) g(q)/fromState2TandTD ==
  data: M input double; xcom input double; c_T_b output double; wHb input double; dxcom input double; dx_b input double; dT output double
function [c_T_b, dT] = centroidalTransformationT_TDot(M,xcom,wHb,dxcom,dx_b)
%#codegen
[c_T_b, dT] = centroidalTransformationT_TDot(xcom,wHb(1:3,4),dxcom,dx_b,M);

== matlab function Subsystem/Dump and visualize/base + dq'/baseVelocity/MATLAB Function ==
  data: JcLeftFoot input double; JcRightFoot input double; activeFeetConstraints input double; y output double; qD input double
function y = fcn(JcLeftFoot,JcRightFoot,activeFeetConstraints,qD)
%#codegen
if sum(activeFeetConstraints) == 2
    Jc = [JcLeftFoot;JcRightFoot];
else
    Jc = JcLeftFoot;
end
y = -pinv(Jc(:,1:6))*Jc(:,7:end)*qD;

== matlab function Subsystem/nonlinearImpedances/nonlinearPosturalGains  ==
  data: qDes input double; nonlinearImpedences output double; q input double; qMin input double; qMax input double; gain parameter double
function nonlinearImpedences = fcn(qDes,q,qMin,qMax,gain)
    %#codegen
    qDes = qDes(:,1);
    impedences_at_0     = gain.impedances;
    increasingRatesImp  = (gain.increasingRatesImp)';
    qTildeMax           = gain.qTildeMax;

    tp =  pi./(2*(qMax-qDes));
    tn = -pi./(2*(qMin-qDes));

    
    qTilde = q - qDes;
            
    nonlinearImpedences = (impedences_at_0'   + increasingRatesImp.*tan(pi.*qTilde./(2*qTildeMax)).^2)';
%                                                increasingRatesImp.*tan((tp.*stepFcn(qTilde) + tn.*stepFcn(-qTilde)).*qTilde).^2)';
                                           
end

function y = stepFcn(x) 
   %#codegen
   y = x > 0; 
end

== matlab function Subsystem/M(q) h(q,dq) g(q)/composingSmoothJacobians ==
  data: constraints input double; JL input double; JR input double; Jc output double; JLNuD input double; JRNuD input double; JcDNuD output double
function [Jc, JcDNuD] = composingSmoothJacobians(constraints,JL,JR, JLNuD,JRNuD)
%#codegen
Jc     = [ JL*constraints(1) ;
           JR*constraints(2)];
       
JcDNuD = [ JLNuD*constraints(1) ;
           JRNuD*constraints(2)];

== matlab function Subsystem/DesValues/Inverse kinematics/iKin correction terms/trajectoryGeneratorCoM ==
  data: lFootPose input double; lFootVel input double; rFootPose input double; rFootVel input double; xC input double; vC input double; qj input double; Dqj input double; iKinFeetCorr output double; CoMRefsDes input double; iKinComCorr output double; iKinPostCorr output double; posturesDes input double; gain parameter double
function [iKinFeetCorr,iKinComCorr,iKinPostCorr]  = fcn(lFootPose,lFootVel,rFootPose,rFootVel,xC,vC,qj,Dqj,CoMRefsDes,posturesDes,gain)
%#codegen

iKinFeetCorr = [-gain.ikin.kp*lFootPose(1:3)-gain.ikin.kd*lFootVel(1:3);
                                            -gain.ikin.kd*lFootVel(4:6);
                -gain.ikin.kp*rFootPose(1:3)-gain.ikin.kd*rFootVel(1:3);
                                            -gain.ikin.kd*rFootVel(4:6)];
                                        
iKinComCorr  = CoMRefsDes(:,3)-gain.ikin.kp*(xC-CoMRefsDes(:,1))-gain.ikin.kd*(vC-CoMRefsDes(:,2));

iKinPostCorr = posturesDes(:,3)-gain.ikin.kp*(qj-posturesDes(:,1))-gain.ikin.kd*(Dqj-posturesDes(:,2));

== matlab function Subsystem/set Base velocity/baseVelocity/MATLAB Function ==
  data: JcLeftFoot input double; JcRightFoot input double; activeFeetConstraints input double; y output double; qD input double; reg parameter double
function y = fcn(JcLeftFoot,JcRightFoot,activeFeetConstraints,qD,reg)
%#codegen

Jc = [ JcLeftFoot*activeFeetConstraints(1);
      JcRightFoot*activeFeetConstraints(2)];

Jcj =  Jc(:,1:6);
pinvJcj = (Jcj')/(Jcj*Jcj' + reg.pinvDamp*eye(size(Jcj,1)));
  
% pinvJcj = pinv(Jc(:,1:6));

y = -pinvJcj*Jc(:,7:end)*qD;
